simulink model "linearizeDrone_motorcmdTostate"  (R2015a)
settings: Solver=ode45  StartTime=0.0  StopTime=10.0  RelTol=1e-3
InitFcn:
  | % load parameters of the default quadrotor
  | disp('Quadrotor parameters loaded by InitFcn')
  | parameters_estimationcontrol %load mdl_quadcopter as well!
undefined symbols (not defined in the file or in its folder): quad, quadEDT
settings Model: Creator=ra  LastModifiedBy=ra

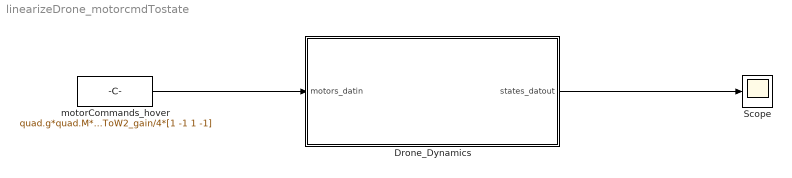
== system linearizeDrone_motorcmdTostate ==
  Drone_Dynamics : Subsystem  AncestorBlock=roblocks/Dynamics/Quadrotor
  Scope : Scope
  motorCommands_hover : Constant  Value=quad.g*quad.M*1/(quad.Ct*quad.rho*quad.A*quad.r^2)*1/quadEDT.motorcommandToW2_gain/4*[1 -1 1 -1]
  wires:
  motorCommands_hover/1 -> Drone_Dynamics/1(motors_datin)
  Drone_Dynamics/1(states_datout) -> Scope/1

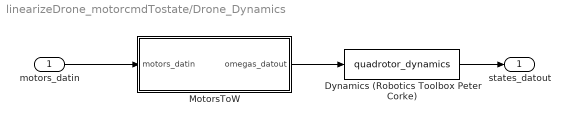
== system linearizeDrone_motorcmdTostate/Drone_Dynamics ==
  motors_datin : Inport
  Dynamics (Robotics Toolbox Peter Corke) : S-Function  FunctionName=quadrotor_dynamics  Parameters=quad
  MotorsToW : Subsystem
  states_datout : Outport
  wires:
  MotorsToW/1(omegas_datout) -> Dynamics (Robotics Toolbox Peter Corke)/1
  motors_datin/1 -> MotorsToW/1(motors_datin)
  Dynamics (Robotics Toolbox Peter Corke)/1 -> states_datout/1

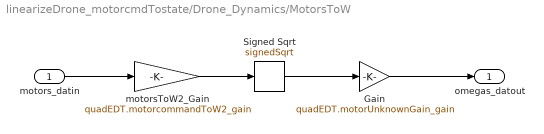
== system linearizeDrone_motorcmdTostate/Drone_Dynamics/MotorsToW ==
  motors_datin : Inport
  Gain : Gain  Gain=quadEDT.motorUnknownGain_gain
  Signed Sqrt : Sqrt  Operator=signedSqrt  SaturateOnIntegerOverflow=on
  motorsToW2_Gain : Gain  Gain=quadEDT.motorcommandToW2_gain
  omegas_datout : Outport
  wires:
  motorsToW2_Gain/1 -> Signed Sqrt/1
  Signed Sqrt/1 -> Gain/1
  motors_datin/1 -> motorsToW2_Gain/1
  Gain/1 -> omegas_datout/1
